simulink model "RBCM_Model"  (R2023b)
settings: Solver=FixedStepAuto  StartTime=0.0  StopTime=10.0  RelTol=1e-3
PreLoadFcn:
  | % NXP_MBDT_S32K3 callback: DO NOT REMOVE
  | mbd_s32k3.common.nxp.model_callbacks.preLoadFcn();
PostLoadFcn:
  | % NXP_MBDT_S32K3 callback: DO NOT REMOVE
  | mbd_s32k3.common.nxp.model_callbacks.postLoadFcn();
InitFcn:
  | % NXP_MBDT_S32K3 callback: DO NOT REMOVE
  | mbd_s32k3.common.nxp.model_callbacks.initFcn();
undefined symbols (not defined in the file or in its folder): AccuFanPwr_hHsd3ch2, BspdPwr_lHsd1ch2, BuzzerPwr_lHsd3ch3, DevicePwr_12v_lHsd1ch1, DevicePwr_hHsd1ch2, DrsPwr_8v_lHsd3ch1, hHsd_Diagnose_AdcBuffer, ILPwr_hHsd1ch1, lHsd_Diagnose_AdcBuffer, LoggerPwr_lHsd1ch3, PumpFan1_hHsd4ch1, PumpFan2_hHsd4ch2, PumpPwr_hHsd3ch1, RGBLED0state, TaillightPwr_lHsd3ch4, TempSensorPwr_lHsd1ch4
libraries: mbd_s32k3_io_library x127, simulink x48, canmsglib x8, mbd_s32k3_communication_library x7, mbd_s32k3_isr_library x6, mbd_s32k3_cdd_library x3, mbd_s32k3_utility_library x1
(part 1 of 9)
settings Model: DataDictionary=RBCM_Model.sldd  Creator=HUAWEI  LastModifiedBy=HUAWEI
settings SolverCC: AutoInsertRateTranBlk=on
settings DataIOCC: ExternalInput=off  InitialState=off  SaveOutput=off  SignalLogging=off  SaveTime=off
settings OptimizationCC: EnhancedBackFolding=on  PassReuseOutputArgsAs=Individual arguments  ZeroExternalMemoryAtStartup=off  ZeroInternalMemoryAtStartup=off  MaxStackSize=64  OptimizeBlockOrder=speed  DifferentSizesBufferReuse=on  OptimizationCustomize=off  EfficientTunableParamExpr=on
settings DebuggingCC: InheritedTsInSrcMsg=none  SingleTaskRateTransMsg=error  ParameterPrecisionLossMsg=none  ParameterTunabilityLossMsg=error  UnconnectedInputMsg=error  UnconnectedOutputMsg=error  UnconnectedLineMsg=error  UnknownTsInhSupMsg=error
settings HardwareCC: ProdBitPerPointer=32  ProdBitPerSizeT=32  ProdBitPerPtrDiffT=32  ProdLargestAtomicInteger=Long  ProdLargestAtomicFloat=Double  ProdWordSize=32  ProdHWDeviceType=ARM Compatible->ARM Cortex
settings SFSimCC: MATLABDynamicMemAlloc=off
settings RTWCC: Description=Embedded Coder  SystemTargetFile=ert.tlc  HardwareBoard=NXP S32K3xx  TemplateMakefile=ert_default_tmf  Toolchain=S32DS GCC  BuildConfiguration=Faster Runs  CheckMdlBeforeBuild=Warning
settings CodeAppCC: ForceParamTrailComments=on  IgnoreCustomStorageClasses=off  OperatorAnnotations=on  SimulinkDataObjDesc=on  SFDataObjDesc=on  InsertBlockDesc=on
settings ERTTargetCC: TargetLangStandard=C99 (ISO)  ExtModeTransport=1  ExtModeMexFile=ext_serial_win32_comm  ERTSrcFileBannerTemplate=mbd_s32k3_ert_code_template.cgt  ERTHdrFileBannerTemplate=mbd_s32k3_ert_code_template.cgt  ERTDataSrcFileTemplate=mbd_s32k3_ert_code_template.cgt  ERTDataHdrFileTemplate=mbd_s32k3_ert_code_template.cgt

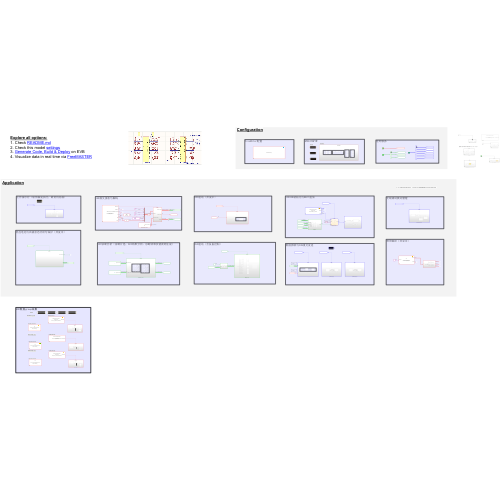
[thumbnail: Simulink's stored preview of the top-level diagram]
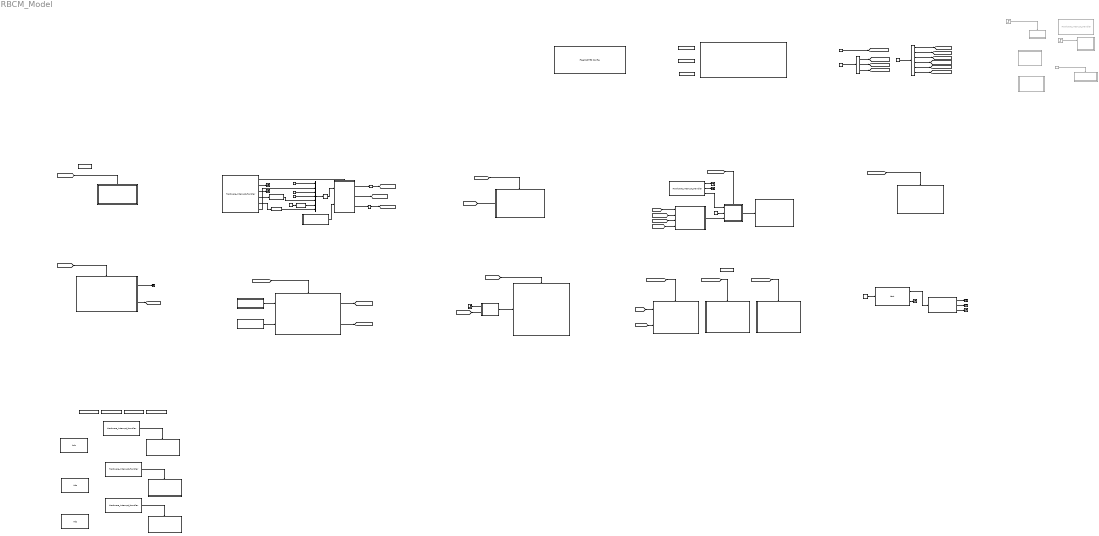
== system RBCM_Model ==
  note: Adc0Group采集
  note: ADC数据group采集
  note: 惯导解析（开发中）
  note: 初始化阶段：逐char接收，判断结束符，结束判收到字符串的ok，有则继续发
      | 通信阶段：只管发，若收转另一条任务链处理
  note: 无线调试模式管理
  note: 低压电池与自板状态分析与保护（开发中）
  note: HSD驱动（含设备控制）
  note: EC800M初始化与MQTT通信
  note: DRS驱动（开发中）
  note: Application
  note: HSD诊断分析（诊断片选、ADC结果分析、诊断结果及错误码生成）
  note: CAN报文接收与解码
  note: 工作指示灯（软件触发执行，最低优先级）
  note: 关于任务调度管理和数据传递：可以考虑采用类似DDS的数据分发服务或相关管理算法
  note: 数据抓取与CAN报文发送
  note: Explore all options:
      | 1. Check README.md
      | 2. Check this model settings
      | 3. Generate Code, Build & Deploy on EVB
      | 4. Visualize data in real time via FreeMASTER
  note: Configuration
  note: Variables
  note: Start ADC Conversions
  note: Hardware Interrupts
  note: Adc1Group采集
  note: Start ADC Conversions
  note: Hardware Interrupts
  note: Adc2Group采集
  note: Start ADC Conversions
  note: Hardware Interrupts
  note: 定时服务
  note: 初始化配置
  note: Variables
  note: Initializations
  note: FreeMster配置
  1000ms1 : simulink/Ports & Subsystems/Function-Call Generator  Priority=4  sample_time=1  numberOfIterations=1  DisallowWideOutput=off
  1000ms4 : simulink/Ports & Subsystems/Function-Call Generator  Priority=4  Commented=on  sample_time=1  numberOfIterations=1  DisallowWideOutput=off
  10ms1 : simulink/Ports & Subsystems/Function-Call Generator  Priority=4  sample_time=0.01  numberOfIterations=1  DisallowWideOutput=off
  4G通信控制状态机1 : Stateflow chart  TreatAsAtomicUnit=on
  50ms1 : simulink/Ports & Subsystems/Function-Call Generator  Priority=4  sample_time=0.05  numberOfIterations=1  DisallowWideOutput=off
  Adc1 : mbd_s32k3_io_library/Adc  api_func=Adc_StartGroupConversion  hw_unit=AdcHwUnit_0  group=Adc1Group_1  channel=hpHSD2_IS_PTD20  threshold_control=AdcThresholdControl_0  power_state=ADC_FULL_POWER  ctu_trigger=AdcHwTrigger_0  ctu_fifo_idx=0  text=<binary blob, 41534 chars, not shown>
      settings: SourceProductName=NXP Model-Based Design Toolbox for S32K3 MCUs
  Adc2 : mbd_s32k3_io_library/Adc  api_func=Adc_StartGroupConversion  hw_unit=AdcHwUnit_0  group=Adc2Group_1  channel=hpHSD2_IS_PTD20  threshold_control=AdcThresholdControl_0  power_state=ADC_FULL_POWER  ctu_trigger=AdcHwTrigger_0  ctu_fifo_idx=0  text=<binary blob, 41534 chars, not shown>
      settings: SourceProductName=NXP Model-Based Design Toolbox for S32K3 MCUs
  Adc3 : mbd_s32k3_io_library/Adc  api_func=Adc_StartGroupConversion  hw_unit=AdcHwUnit_0  group=Adc0Group_1  channel=hpHSD2_IS_PTD20  threshold_control=AdcThresholdControl_0  power_state=ADC_FULL_POWER  ctu_trigger=AdcHwTrigger_0  ctu_fifo_idx=0  text=<binary blob, 41534 chars, not shown>
      settings: SourceProductName=NXP Model-Based Design Toolbox for S32K3 MCUs
  Bitwise AND : simulink/Logic and Bit Operations/Bitwise Operator  logicop=AND  UseBitMask=on  BitMask=0x1fffffff  BitMaskRealWorld=Stored Integer
      settings: LibrarySourceBlock=|
      | simulink/Quick Insert/Logic and Bit
      | Operations/Bitwise AND
  Bus Creator1 : BusCreator  Inputs=7  OutDataTypeStr=Bus: Bus_CAN_RX_MESSAG  NonVirtualBus=on
  Constant : Constant
  Constant1 : Constant  Value=41  OutDataTypeStr=uint32
  Constant13 : Constant  Value=0  OutDataTypeStr=uint8
  Constant2 : Constant  OutDataTypeStr=uint8
  Constant4 : Constant  OutMax=[255]  OutDataTypeStr=uint8
  Constant6 : Constant  Value=0  OutDataTypeStr=uint8
  Data Store Memory1 : DataStoreMemory  DataStoreName=Adc0Group1_ResultBuffer  ReadBeforeWriteMsg=warning  WriteAfterWriteMsg=warning  WriteAfterReadMsg=warning  InitialValue=[0, 0, 0, 0, 0, 0]  ShowAdditionalParam=off  OutDataTypeStr=uint16
  Data Store Memory2 : DataStoreMemory  DataStoreName=Temp_AdcBuffer  WriteAfterWriteMsg=warning  ShowAdditionalParam=off  OutDataTypeStr=uint16
  Data Store Memory3 : DataStoreMemory  DataStoreName=can_id  ReadBeforeWriteMsg=warning  WriteAfterWriteMsg=warning  WriteAfterReadMsg=warning  ShowAdditionalParam=off  OutDataTypeStr=uint32
  Data Store Memory4 : DataStoreMemory  DataStoreName=Bats_Monitor_AdcBuffer  WriteAfterWriteMsg=warning  InitialValue=[0 0]  ShowAdditionalParam=off  OutDataTypeStr=uint16
  Data Store Memory5 : DataStoreMemory  DataStoreName=hHsd_Diagnose_AdcBuffer  WriteAfterWriteMsg=warning  InitialValue=[0 0 0 0 0 0]  ShowAdditionalParam=off  OutDataTypeStr=uint16
  Data Store Memory6 : DataStoreMemory  DataStoreName=lHsd_Diagnose_AdcBuffer  WriteAfterWriteMsg=warning  InitialValue=[0 0 0 0 0]  ShowAdditionalParam=off  OutDataTypeStr=uint16
  Data Store Memory7 : DataStoreMemory  DataStoreName=Adc1Group1_ResultBuffer  ReadBeforeWriteMsg=warning  WriteAfterWriteMsg=warning  WriteAfterReadMsg=warning  InitialValue=[0, 0, 0]  ShowAdditionalParam=off  OutDataTypeStr=uint16
  Data Store Memory8 : DataStoreMemory  DataStoreName=Adc2Group1_ResultBuffer  ReadBeforeWriteMsg=warning  WriteAfterWriteMsg=warning  WriteAfterReadMsg=warning  InitialValue=[0, 0, 0, 0, 0]  ShowAdditionalParam=off  OutDataTypeStr=uint16
  Data Type Conversion2 : DataTypeConversion  OutDataTypeStr=double  SaturateOnIntegerOverflow=off  RndMeth=Floor
  Delay : Delay  DelayLength=1
  FreeMASTER Config : mbd_s32k3_utility_library/FreeMASTER blocks/FreeMASTER Config  connection_type=Serial  instance=LPUART_6  baudrate=115200  isr_prio=5  cantxid=0x7aa  cantxidext=on  cantxobj=5  canrxid=0x7aa  canrxidext=on  canrxobj=5  mode=Short Interrupt  scope_use=1  scope_max_vars=8  automatic_buff_size=on  buff_size=255  default_rfifo_size=on  rfifo_size=32  text=This peripheral is not configured in the project associated to the model.
      settings: SourceProductName=NXP Model-Based Design Toolbox for S32K3 MCUs
  Function-Call Split : FunctionCallSplit  IconShape=distinctive  NumOutputPorts=6  OutputPortLayout=default
  Function-Call Split1 : FunctionCallSplit  IconShape=distinctive  NumOutputPorts=3  OutputPortLayout=default
  HSD诊断分析子系统 : Subsystem
  HSD诊断数据抓取与发送(不启用) : Subsystem  Commented=on
  HSD驱动子系统 : Subsystem
  Hardware_Interrupt_Handler : mbd_s32k3_isr_library/Hardware_Interrupt_Handler  blockCbk=0  irqGroup=Uart  irqHandlers=MBDT_Uart_Callback  irqSim=off  text=<binary blob, 5810 chars, not shown>
      settings: SourceProductName=NXP Model-Based Design Toolbox for S32K3 MCUs
  Hardware_Interrupt_Handler1 : mbd_s32k3_isr_library/Hardware_Interrupt_Handler  blockCbk=0  irqGroup=Adc  irqHandlers=Adc_Adc0Group1Notification  irqSim=off  text=<binary blob, 41534 chars, not shown>
      settings: SourceProductName=NXP Model-Based Design Toolbox for S32K3 MCUs
  Hardware_Interrupt_Handler2 : mbd_s32k3_isr_library/Hardware_Interrupt_Handler  blockCbk=0  irqGroup=Adc  irqHandlers=Adc_Adc1Group1Notification  irqSim=off  text=<binary blob, 41534 chars, not shown>
      settings: SourceProductName=NXP Model-Based Design Toolbox for S32K3 MCUs
  Hardware_Interrupt_Handler4 : mbd_s32k3_isr_library/Hardware_Interrupt_Handler  blockCbk=0  irqGroup=Can  irqHandlers=CanIf_RxIndication  irqSim=off  text=|
      | CanConfigSet - CanConfigSet 
      | CanConfigSet/CanController - CanController_0 
      | CanConfigSet/CanController_0/CanAutoBusOffRecovery - false 
      | CanConfigSet/CanController_0/CanBusoffProcessing - POLLING 
      | CanConfigSet/CanController_0/CanControllerActivation - true 
      | CanConfigSet/CanController_0/CanControllerBaseAddress - 0 
      | CanConfigSet/CanController_0/CanControllerBaudrateConfig - CanControllerBaudrateConfig_0 
      | CanConfigSet/CanController_0/CanControllerBaudrateConfig_0/CanAdvancedSetting - false 
      | CanConfigSet/CanController_0/CanControllerBaudrateConfig_0/CanBaudrateTypeSuport - NORMAL_CBT 
      | CanConfigSet/CanController_0/CanControllerBaudrateConfig_0/CanBusLength - 40 
      | CanConfigSet/CanController_0/CanControllerBaudrateConfig_0/CanControllerBaudRate - 500.0 
      | CanConfigSet/CanController_0/CanControllerBaudrateConfig_0/CanControllerBaudRateConfigID - 0 
      | CanConfigSet/CanController_0/CanControllerBaudrateConfig_0/CanControllerFdBaudrateConfig - CanControllerFdBaudrateConfig 
      | CanConfigSet/CanController_0/CanControllerBaudrateConfig_0/CanControllerFdBaudrateConfig/CanControllerFdBaudRate - 2000 
      | CanConfigSet/CanController_0/CanControllerBaudrateConfig_0/CanControllerFdBaudrateConfig/CanControllerFdPrescaller - 2 
      | CanConfigSet/CanController_0/CanControllerBaudrateConfig_0/CanControllerFdBaudrateConfig/CanControllerFdSyncSeg - 1 
      | CanConfigSet/CanController_0/CanControllerBaudrateConfig_0/CanControllerFdBaudrateConfig/CanControllerPrescallerAlternateFd - 1 
      | CanConfigSet/CanController_0/CanControllerBaudrateConfig_0/CanControllerFdBaudrateConfig/CanControllerPropSeg - 5 
      | CanConfigSet/CanController_0/CanControllerBaudrateConfig_0/CanControllerFdBaudrateConfig/CanControllerSeg1 - 2 
      | CanConfigSet/CanController_0/CanControllerBaudrateConfig_0/CanControllerFdBaudrateConfig/CanControllerSeg2 - 2 
      | CanConfigSet/CanController_0/CanControllerBaudrateConfig_0/CanControllerFdBaudrateConfig/CanControllerSyncJumpWidth - 2 
      | CanConfigSet/CanController_0/CanControllerBaudrateConfig_0/CanControllerFdBaudrateConfig/CanControllerTxBitRateSwitch - true 
      | CanConfigSet/CanController_0/CanControllerBaudrateConfig_0/CanControllerFdBaudrateConfig/Index - 0 
      | CanConfigSet/CanController_0/CanControllerBaudrateConfig_0/CanControllerPrescaller - 2 
      | CanConfigSet/CanController_0/CanControllerBaudrateConfig_0/CanControllerPrescallerAlternate - 10 
      | CanConfigSet/CanController_0/CanControllerBaudrateConfig_0/CanControllerPropSeg - 11 
      | CanConfigSet/CanController_0/CanControllerBaudrateConfig_0/CanControllerSeg1 - 18 
      | CanConfigSet/CanController_0/CanControllerBaudrateConfig_0/CanControllerSeg2 - 10 
      | CanConfigSet/CanController_0/CanControllerBaudrateConfig_0/CanControllerSyncJumpWidth - 10 
      | CanConfigSet/CanController_0/CanControllerBaudrateConfig_0/CanControllerSyncSeg - 1 
      | CanConfigSet/CanController_0/CanControllerBaudrateConfig_0/CanPropDelayTranceiver - 150.0 
      | CanConfigSet/CanController_0/CanControllerBaudrateConfig_0/CanTxArbitrationStartDelay - 12 
      | CanConfigSet/CanController_0/CanControllerBaudrateConfig_0/Index - 0 
      | CanConfigSet/CanController_0/CanControllerDefaultBaudrate - /Can_43_FLEXCAN/Can/CanConfigSet/CanController_0/CanControllerBaudrateConfig_0 
      | CanConfigSet/CanController_0/CanControllerEdgeFilter - false 
      | CanConfigSet/CanController_0/CanControllerFdISO - true 
      | CanConfigSet/CanController_0/CanControllerId - 0 
      | CanConfigSet/CanController_0/CanControllerPrExcEn - false 
      | CanConfigSet/CanController_0/CanCpuClockRef - /Mcu/Mcu/McuModuleConfiguration/McuClockSettingConfig_0/FLEXCAN_PE_CLK0_2 
      | CanConfigSet/CanController_0/CanCpuClockRefAlternate - /Mcu/Mcu/McuModuleConfiguration/McuClockSettingConfig_0/FLEXCAN_PE_CLK0_2 
      | CanConfigSet/CanController_0/CanHwChannel - FLEXCAN_0 
      | CanConfigSet/CanController_0/CanLoopBackMode - false 
      | CanConfigSet/CanController_0/CanRamBlock - CanRamBlock 
      | CanConfigSet/CanController_0/CanRamBlock/CanRamBlockUnified - CanRamBlockUnified 
      | CanConfigSet/CanController_0/CanRamBlock/CanRamBlockUnified/CanBlockUnifiedPayloadLength - CAN_16_BYTES_PAYLOAD 
      | CanConfigSet/CanController_0/CanRamBlock/Choice - CanRamBlockUnified 
      | CanConfigSet/CanController_0/CanRamBlock/Index - 0 
      | CanConfigSet/CanController_0/CanRxFiFo - CanRxFiFo 
      | CanConfigSet/CanController_0/CanRxFiFo/CanEnhanceFiFo - CanRxFiFo 
      | CanConfigSet/CanController_0/CanRxFiFo/CanRxFiFo/CanEnhanceFiFoDmaEnable - false 
      | CanConfigSet/CanController_0/CanRxFiFo/CanRxFiFo/CanEnhancedSchemeType - MASK_FILTER_SCHEME 
      | CanConfigSet/CanController_0/CanRxFiFo/CanRxFiFo/CanFiFoDmaErrorNotif - NULL_PTR 
      | CanConfigSet/CanController_0/CanRxFiFo/CanRxFiFo/CanFiFoOverflowNotif - MBDT_FlexCAN0_FifoOverflowNotif 
      | CanConfigSet/CanController_0/CanRxFiFo/CanRxFiFo/NumberMBTransferDMA - 1 
      | CanConfigSet/CanController_0/CanRxFiFo/Choice - CanEnhanceFiFo 
      | CanConfigSet/CanController_0/CanRxFiFo/Index - 0 
      | CanConfigSet/CanController_0/CanRxProcessing - MIXED 
      | CanConfigSet/CanController_0/CanTrippleSamplingEnable - false 
      | CanConfigSet/CanController_0/CanTxProcessing - MIXED 
      | CanConfigSet/CanController_0/CanWakeupFunctionalityAPI - false 
      | CanConfigSet/CanController_0/CanWakeupProcessing - POLLING 
      | CanConfigSet/CanController_0/CanWakeupSupport - false 
      | CanConfigSet/CanController_0/Index - 0 
      | CanConfigSet/CanHardwareObject - CanHardwareObject_Can0_Rx_Ext_Interrupt CanHardwareObject_Can0_Rx_FIFO CanHardwareObject_Can0_Rx_Std_Polling CanHardwareObject_Can0_Tx_Interrupt CanHardwareObject_Can0_Tx_Polling 
      | CanConfigSet/CanHardwareObject_Can0_Rx_Ext_Interrupt/CanControllerRef - /Can_43_FLEXCAN/Can/CanConfigSet/CanController_0 
      | CanConfigSet/CanHardwareObject_Can0_Rx_Ext_Interrupt/CanHandleType - BASIC 
      | CanConfigSet/CanHardwareObject_Can0_Rx_Ext_Interrupt/CanHardwareObjectUsesPolling - false 
      | CanConfigSet/CanHardwareObject_Can0_Rx_Ext_Interrupt/CanHwFilter - CanHwFilter_0 
      | CanConfigSet/CanHardwareObject_Can0_Rx_Ext_Interrupt/CanHwFilter_0/CanHwFilterCode - 0 
      | CanConfigSet/CanHardwareObject_Can0_Rx_Ext_Interrupt/CanHwFilter_0/CanHwFilterMask - 0 
      | CanConfigSet/CanHardwareObject_Can0_Rx_Ext_Interrupt/CanHwFilter_0/Index - 0 
      | CanConfigSet/CanHardwareObject_Can0_Rx_Ext_Interrupt/CanHwObjectCount - 1 
      | CanConfigSet/CanHardwareObject_Can0_Rx_Ext_Interrupt/CanIdType - EXTENDED 
      | CanConfigSet/CanHardwareObject_Can0_Rx_Ext_Interrupt/CanObjectId - 2 
      | CanConfigSet/CanHardwareObject_Can0_Rx_Ext_Interrupt/CanObjectType - RECEIVE 
      | CanConfigSet/CanHardwareObject_Can0_Rx_Ext_Interrupt/Index - 2 
      | CanConfigSet/CanHardwareObject_Can0_Rx_FIFO/CanControllerRef - /Can_43_FLEXCAN/Can/CanConfigSet/CanController_0 
      | CanConfigSet/CanHardwareObject_Can0_Rx_FIFO/CanHandleType - BASIC 
      | CanConfigSet/CanHardwareObject_Can0_Rx_FIFO/CanHardwareObjectUsesPolling - false 
      | CanConfigSet/CanHardwareObject_Can0_Rx_FIFO/CanHwFilter - CanHwFilter_0 CanHwFilter_1 CanHwFilter_2 CanHwFilter_3 CanHwFilter_4 CanHwFilter_5 CanHwFilter_6 CanHwFilter_7 
      | CanConfigSet/CanHardwareObject_Can0_Rx_FIFO/CanHwFilter_0/CanHwFilterCode - 1008 
      | CanConfigSet/CanHardwareObject_Can0_Rx_FIFO/CanHwFilter_0/CanHwFilterMask - 536870911 
      | CanConfigSet/CanHardwareObject_Can0_Rx_FIFO/CanHwFilter_0/Index - 0 
      | CanConfigSet/CanHardwareObject_Can0_Rx_FIFO/CanHwFilter_1/CanHwFilterCode - 1009 
      | CanConfigSet/CanHardwareObject_Can0_Rx_FIFO/CanHwFilter_1/CanHwFilterMask - 536870911 
      | CanConfigSet/CanHardwareObject_Can0_Rx_FIFO/CanHwFilter_1/Index - 1 
      | CanConfigSet/CanHardwareObject_Can0_Rx_FIFO/CanHwFilter_2/CanHwFilterCode - 1010 
      | CanConfigSet/CanHardwareObject_Can0_Rx_FIFO/CanHwFilter_2/CanHwFilterMask - 536870911 
      | CanConfigSet/CanHardwareObject_Can0_Rx_FIFO/CanHwFilter_2/Index - 2 
      | CanConfigSet/CanHardwareObject_Can0_Rx_FIFO/CanHwFilter_3/CanHwFilterCode - 1011 
      | CanConfigSet/CanHardwareObject_Can0_Rx_FIFO/CanHwFilter_3/CanHwFilterMask - 536870911 
      | CanConfigSet/CanHardwareObject_Can0_Rx_FIFO/CanHwFilter_3/Index - 3 
      | CanConfigSet/CanHardwareObject_Can0_Rx_FIFO/CanHwFilter_4/CanHwFilterCode - 1012 
      | CanConfigSet/CanHardwareObject_Can0_Rx_FIFO/CanHwFilter_4/CanHwFilterMask - 536870911 
      | CanConfigSet/CanHardwareObject_Can0_Rx_FIFO/CanHwFilter_4/Index - 4 
      | CanConfigSet/CanHardwareObject_Can0_Rx_FIFO/CanHwFilter_5/CanHwFilterCode - 1013 
      | CanConfigSet/CanHardwareObject_Can0_Rx_FIFO/CanHwFilter_5/CanHwFilterMask - 536870911 
      | CanConfigSet/CanHardwareObject_Can0_Rx_FIFO/CanHwFilter_5/Index - 5 
      | CanConfigSet/CanHardwareObject_Can0_Rx_FIFO/CanHwFilter_6/CanHwFilterCode - 1014 
      | CanConfigSet/CanHardwareObject_Can0_Rx_FIFO/CanHwFilter_6/CanHwFilterMask - 536870911 
      | CanConfigSet/CanHardwareObject_Can0_Rx_FIFO/CanHwFilter_6/Index - 6 
      | CanConfigSet/CanHardwareObject_Can0_Rx_FIFO/CanHwFilter_7/CanHwFilterCode - 1015 
      | CanConfigSet/CanHardwareObject_Can0_Rx_FIFO/CanHwFilter_7/CanHwFilterMask - 536870911 
      | CanConfigSet/CanHardwareObject_Can0_Rx_FIFO/CanHwFilter_7/Index - 7 
      | CanConfigSet/CanHardwareObject_Can0_Rx_FIFO/CanHwObjectCount - 6 
      | CanConfigSet/CanHardwareObject_Can0_Rx_FIFO/CanIdType - EXTENDED 
      | CanConfigSet/CanHardwareObject_Can0_Rx_FIFO/CanObjectId - 0 
      | CanConfigSet/CanHardwareObject_Can0_Rx_FIFO/CanObjectType - RECEIVE 
      | CanConfigSet/CanHardwareObject_Can0_Rx_FIFO/Index - 0 
      | CanConfigSet/CanHardwareObject_Can0_Rx_Std_Polling/CanControllerRef - /Can_43_FLEXCAN/Can/CanConfigSet/CanController_0 
      | CanConfigSet/CanHardwareObject_Can0_Rx_Std_Polling/CanHandleType - BASIC 
      | CanConfigSet/CanHardwareObject_Can0_Rx_Std_Polling/CanHardwareObjectUsesPolling - true 
      | CanConfigSet/CanHardwareObject_Can0_Rx_Std_Polling/CanHwFilter - CanHwFilter_0 
      | CanConfigSet/CanHardwareObject_Can0_Rx_Std_Polling/CanHwFilter_0/CanHwFilterCode - 0 
      | CanConfigSet/CanHardwareObject_Can0_Rx_Std_Polling/CanHwFilter_0/CanHwFilterMask - 0 
      | CanConfigSet/CanHardwareObject_Can0_Rx_Std_Polling/CanHwFilter_0/Index - 0 
      | CanConfigSet/CanHardwareObject_Can0_Rx_Std_Polling/CanHwObjectCount - 1 
      | CanConfigSet/CanHardwareObject_Can0_Rx_Std_Polling/CanIdType - STANDARD 
      | CanConfigSet/CanHardwareObject_Can0_Rx_Std_Polling/CanMainFunctionRWPeriodRef - /Can_43_FLEXCAN/Can/CanGeneral/CanMainFunctionRWPeriods_0 
      | CanConfigSet/CanHardwareObject_Can0_Rx_Std_Polling/CanObjectId - 1 
      | CanConfigSet/CanHardwareObject_Can0_Rx_Std_Polling/CanObjectType - RECEIVE 
      | CanConfigSet/CanHardwareObject_Can0_Rx_Std_Polling/Index - 1 
      | CanConfigSet/CanHardwareObject_Can0_Tx_Interrupt/CanControllerRef - /Can_43_FLEXCAN/Can/CanConfigSet/CanController_0 
      | CanConfigSet/CanHardwareObject_Can0_Tx_Interrupt/CanHandleType - BASIC 
      | CanConfigSet/CanHardwareObject_Can0_Tx_Interrupt/CanHardwareObjectUsesPolling - false 
      | CanConfigSet/CanHardwareObject_Can0_Tx_Interrupt/CanHwObjectCount - 1 
      | CanConfigSet/CanHardwareObject_Can0_Tx_Interrupt/CanIdType - MIXED 
      | CanConfigSet/CanHardwareObject_Can0_Tx_Interrupt/CanObjectId - 4 
      | CanConfigSet/CanHardwareObject_Can0_Tx_Interrupt/CanObjectType - TRANSMIT 
      | CanConfigSet/CanHardwareObject_Can0_Tx_Interrupt/Index - 4 
      | CanConfigSet/CanHardwareObject_Can0_Tx_Polling/CanControllerRef - /Can_43_FLEXCAN/Can/CanConfigSet/CanController_0 
      | CanConfigSet/CanHardwareObject_Can0_Tx_Polling/CanHandleType - BASIC 
      | CanConfigSet/CanHardwareObject_Can0_Tx_Polling/CanHardwareObjectUsesPolling - true 
      | CanConfigSet/CanHardwareObject_Can0_Tx_Polling/CanHwObjectCount - 1 
      | CanConfigSet/CanHardwareObject_Can0_Tx_Polling/CanIdType - MIXED 
      | CanConfigSet/CanHardwareObject_Can0_Tx_Polling/CanMainFunctionRWPeriodRef - /Can_43_FLEXCAN/Can/CanGeneral/CanMainFunctionRWPeriods_0 
      | CanConfigSet/CanHardwareObject_Can0_Tx_Polling/CanObjectId - 3 
      | CanConfigSet/CanHardwareObject_Can0_Tx_Polling/CanObjectType - TRANSMIT 
      | CanConfigSet/CanHardwareObject_Can0_Tx_Polling/Index - 3 
      | CanGeneral - CanGeneral 
      | CanGeneral/CanApiEnableMbAbort - true 
      | CanGeneral/CanDevErrorDetect - true 
      | CanGeneral/CanEnableDualClockMode - false 
      | CanGeneral/CanEnableSecurityEventReporting - false 
      | CanGeneral/CanEnableUserModeSupport - false 
      | CanGeneral/CanGlobalTimeSupport - false 
      | CanGeneral/CanIndex - 0 
      | CanGeneral/CanMBCountExtensionSupport - false 
      | CanGeneral/CanMainFunctionModePeriod - 0.001 
      | CanGeneral/CanMainFunctionRWPeriods - CanMainFunctionRWPeriods_0 
      | CanGeneral/CanMainFunctionRWPeriods_0/CanMainFunctionPeriod - 0.001 
      | CanGeneral/CanMainFunctionRWPeriods_0/Index - 0 
      | CanGeneral/CanMultiPartitionSupport - false 
      | CanGeneral/CanMultiplexedTransmission - true 
      | CanGeneral/CanSetBaudrateApi - true 
      | CanGeneral/CanTimeoutDuration - 1.0 
      | CanGeneral/CanTimeoutMethod - OSIF_COUNTER_DUMMY 
      | CanGeneral/CanVersionInfoApi - true 
      | CommonPublishedInformation - CommonPublishedInformation 
      | CommonPublishedInformation/ArReleaseMajorVersion - 4 
      | CommonPublishedInformation/ArReleaseMinorVersion - 7 
      | CommonPublishedInformation/ArReleaseRevisionVersion - 0 
      | CommonPublishedInformation/ModuleId - 80 
      | CommonPublishedInformation/SwMajorVersion - 3 
      | CommonPublishedInformation/SwMinorVersion - 0 
      | CommonPublishedInformation/SwPatchVersion - 0 
      | CommonPublishedInformation/VendorApiInfix - FLEXCAN 
      | CommonPublishedInformation/VendorId - 43 
      | IMPLEMENTATION-CONFIG-VARIANT - VARIANT-POST-BUILD 
      | POST_BUILD_VARIANT_USED - true
      settings: SourceProductName=NXP Model-Based Design Toolbox for S32K3 MCUs
  Hardware_Interrupt_Handler5 : mbd_s32k3_isr_library/Hardware_Interrupt_Handler  blockCbk=0  irqGroup=Adc  irqHandlers=Adc_Adc2Group1Notification  irqSim=off  text=<binary blob, 41534 chars, not shown>
      settings: SourceProductName=NXP Model-Based Design Toolbox for S32K3 MCUs
  Hardware_Interrupt_Handler6 : mbd_s32k3_isr_library/Hardware_Interrupt_Handler  Commented=on  blockCbk=0  irqGroup=Pwm  irqHandlers=PwmChannel_0_Callback  irqSim=off  text=|
      | CommonPublishedInformation - CommonPublishedInformation Pwm 
      | CommonPublishedInformation/ArReleaseMajorVersion - 4 
      | CommonPublishedInformation/ArReleaseMinorVersion - 4 
      | CommonPublishedInformation/ArReleaseRevisionVersion - 0 
      | CommonPublishedInformation/ModuleId - 121 
      | CommonPublishedInformation/SwMajorVersion - 2 
      | CommonPublishedInformation/SwMinorVersion - 0 
      | CommonPublishedInformation/SwPatchVersion - 0 
      | CommonPublishedInformation/VendorId - 43 
      | IMPLEMENTATION-CONFIG-VARIANT - VARIANT-POST-BUILD 
      | POST_BUILD_VARIANT_USED - true 
      | PwmChannel - PwmChannel_0 PwmChannel_1 PwmChannel_2 PwmChannel_3 PwmChannel_4 PwmChannel_5 PwmChannel_6 PwmChannel_7 PwmChannel_8 
      | PwmChannel_0/Index - 0 
      | PwmChannel_0/PwmChannelId - 0 
      | PwmChannel_0/PwmDutycycleDefault - 2048 
      | PwmChannel_0/PwmHwChannel - /Pwm/Pwm/PwmChannelConfigSet/PwmEmios_0/PwmEmiosChannels_9 
      | PwmChannel_0/PwmIdleState - PWM_LOW 
      | PwmChannel_0/PwmMcuClockReferencePoint - /Mcu/Mcu/McuModuleConfiguration/McuClockSettingConfig_0/CORE_CLK 
      | PwmChannel_0/PwmNotification - PwmChannel_0_Callback 
      | PwmChannel_0/PwmPeriodDefault - 16000.0 
      | PwmChannel_0/PwmPeriodInTicks - true 
      | PwmChannel_0/PwmPolarity - PWM_HIGH 
      | PwmChannel_1/Index - 1 
      | PwmChannel_1/PwmChannelId - 1 
      | PwmChannel_1/PwmDutycycleDefault - 2048 
      | PwmChannel_1/PwmHwChannel - /Pwm/Pwm/PwmChannelConfigSet/PwmEmios_0/PwmEmiosChannels_17 
      | PwmChannel_1/PwmIdleState - PWM_LOW 
      | PwmChannel_1/PwmMcuClockReferencePoint - /Mcu/Mcu/McuModuleConfiguration/McuClockSettingConfig_0/CORE_CLK 
      | PwmChannel_1/PwmNotification - PwmChannel_1_Callback 
      | PwmChannel_1/PwmPeriodDefault - 16000.0 
      | PwmChannel_1/PwmPeriodInTicks - true 
      | PwmChannel_1/PwmPolarity - PWM_HIGH 
      | PwmChannel_2/Index - 2 
      | PwmChannel_2/PwmChannelId - 2 
      | PwmChannel_2/PwmDutycycleDefault - 0 
      | PwmChannel_2/PwmHwChannel - /Pwm/Pwm/PwmChannelConfigSet/PwmEmios_1/PwmEmiosChannels_19 
      | PwmChannel_2/PwmIdleState - PWM_LOW 
      | PwmChannel_2/PwmMcuClockReferencePoint - /Mcu/Mcu/McuModuleConfiguration/McuClockSettingConfig_0/CORE_CLK 
      | PwmChannel_2/PwmNotification - PwmChannel_2_Callback 
      | PwmChannel_2/PwmPeriodDefault - 16000.0 
      | PwmChannel_2/PwmPeriodInTicks - true 
      | PwmChannel_2/PwmPolarity - PWM_HIGH 
      | PwmChannel_3/Index - 3 
      | PwmChannel_3/PwmChannelId - 3 
      | PwmChannel_3/PwmDutycycleDefault - 0 
      | PwmChannel_3/PwmHwChannel - /Pwm/Pwm/PwmChannelConfigSet/PwmEmios_1/PwmEmiosChannels_20 
      | PwmChannel_3/PwmIdleState - PWM_LOW 
      | PwmChannel_3/PwmMcuClockReferencePoint - /Mcu/Mcu/McuModuleConfiguration/McuClockSettingConfig_0/CORE_CLK 
      | PwmChannel_3/PwmNotification - PwmChannel_3_Callback 
      | PwmChannel_3/PwmPeriodDefault - 16000.0 
      | PwmChannel_3/PwmPeriodInTicks - true 
      | PwmChannel_3/PwmPolarity - PWM_HIGH 
      | PwmChannel_4/Index - 4 
      | PwmChannel_4/PwmChannelId - 4 
      | PwmChannel_4/PwmDutycycleDefault - 0 
      | PwmChannel_4/PwmHwChannel - /Pwm/Pwm/PwmChannelConfigSet/PwmEmios_1/PwmEmiosChannels_0 
      | PwmChannel_4/PwmIdleState - PWM_LOW 
      | PwmChannel_4/PwmMcuClockReferencePoint - /Mcu/Mcu/McuModuleConfiguration/McuClockSettingConfig_0/CORE_CLK 
      | PwmChannel_4/PwmNotification - PwmChannel_4_Callback 
      | PwmChannel_4/PwmPeriodDefault - 16000.0 
      | PwmChannel_4/PwmPeriodInTicks - true 
      | PwmChannel_4/PwmPolarity - PWM_HIGH 
      | PwmChannel_5/Index - 5 
      | PwmChannel_5/PwmChannelId - 5 
      | PwmChannel_5/PwmDutycycleDefault - 0 
      | PwmChannel_5/PwmHwChannel - /Pwm/Pwm/PwmChannelConfigSet/PwmEmios_1/PwmEmiosChannels_1 
      | PwmChannel_5/PwmIdleState - PWM_LOW 
      | PwmChannel_5/PwmMcuClockReferencePoint - /Mcu/Mcu/McuModuleConfiguration/McuClockSettingConfig_0/CORE_CLK 
      | PwmChannel_5/PwmNotification - PwmChannel_5_Callback 
      | PwmChannel_5/PwmPeriodDefault - 16000.0 
      | PwmChannel_5/PwmPeriodInTicks - true 
      | PwmChannel_5/PwmPolarity - PWM_HIGH 
      | PwmChannel_6/Index - 6 
      | PwmChannel_6/PwmChannelId - 6 
      | PwmChannel_6/PwmDutycycleDefault - 0 
      | PwmChannel_6/PwmHwChannel - /Pwm/Pwm/PwmChannelConfigSet/PwmEmios_1/PwmEmiosChannels_21 
      | PwmChannel_6/PwmIdleState - PWM_LOW 
      | PwmChannel_6/PwmMcuClockReferencePoint - /Mcu/Mcu/McuModuleConfiguration/McuClockSettingConfig_0/CORE_CLK 
      | PwmChannel_6/PwmNotification - PwmChannel_6_Callback 
      | PwmChannel_6/PwmPeriodDefault - 16000.0 
      | PwmChannel_6/PwmPeriodInTicks - true 
      | PwmChannel_6/PwmPolarity - PWM_HIGH 
      | PwmChannel_7/Index - 7 
      | PwmChannel_7/PwmChannelId - 7 
      | PwmChannel_7/PwmDutycycleDefault - 0 
      | PwmChannel_7/PwmHwChannel - /Pwm/Pwm/PwmChannelConfigSet/PwmEmios_1/PwmEmiosChannels_22 
      | PwmChannel_7/PwmIdleState - PWM_LOW 
      | PwmChannel_7/PwmMcuClockReferencePoint - /Mcu/Mcu/McuModuleConfiguration/McuClockSettingConfig_0/CORE_CLK 
      | PwmChannel_7/PwmNotification - PwmChannel_7_Callback 
      | PwmChannel_7/PwmPeriodDefault - 16000.0 
      | PwmChannel_7/PwmPeriodInTicks - true 
      | PwmChannel_7/PwmPolarity - PWM_HIGH 
      | PwmChannel_8/Index - 8 
      | PwmChannel_8/PwmChannelId - 8 
      | PwmChannel_8/PwmDutycycleDefault - 0 
      | PwmChannel_8/PwmHwChannel - /Pwm/Pwm/PwmChannelConfigSet/PwmEmios_2/PwmEmiosChannels_7 
      | PwmChannel_8/PwmIdleState - PWM_LOW 
      | PwmChannel_8/PwmMcuClockReferencePoint - /Mcu/Mcu/McuModuleConfiguration/McuClockSettingConfig_0/CORE_CLK 
      | PwmChannel_8/PwmNotification - PwmChannel_8_Callback 
      | PwmChannel_8/PwmPeriodDefault - 40000 
      | PwmChannel_8/PwmPeriodInTicks - true 
      | PwmChannel_8/PwmPolarity - PWM_HIGH 
      | PwmConfigurationOfOptApiServices - PwmConfigurationOfOptApiServices 
      | PwmConfigurationOfOptApiServices/PwmDeInitApi - true 
      | PwmConfigurationOfOptApiServices/PwmEmiosFastUpdateApi - true 
      | PwmConfigurationOfOptApiServices/PwmEnableMaskOutputs - false 
      | PwmConfigurationOfOptApiServices/PwmGetChannelStateApi - true 
      | PwmConfigurationOfOptApiServices/PwmGetOutputState - true 
      | PwmConfigurationOfOptApiServices/PwmSetChannelDeadTime - true 
      | PwmConfigurationOfOptApiServices/PwmSetChannelOutputApi - true 
      | PwmConfigurationOfOptApiServices/PwmSetCounterBusApi - true 
      | PwmConfigurationOfOptApiServices/PwmSetDutyCycle - true 
      | PwmConfigurationOfOptApiServices/PwmSetDutyCycle_NoUpdate - false 
      | PwmConfigurationOfOptApiServices/PwmSetDutyPhaseShift - false 
      | PwmConfigurationOfOptApiServices/PwmSetOutputToIdle - true 
      | PwmConfigurationOfOptApiServices/PwmSetPeriodAndDuty - true 
      | PwmConfigurationOfOptApiServices/PwmSetPeriodAndDuty_NoUpdate - false 
      | PwmConfigurationOfOptApiServices/PwmSetTriggerDelayApi - true 
      | PwmConfigurationOfOptApiServices/PwmVersionInfoApi - true 
      | PwmEmios - PwmEmios_0 PwmEmios_1 PwmEmios_2 
      | PwmEmios_0/Index - 0 
      | PwmEmios_0/PwmEmiosChannels - PwmEmiosChannels_17 PwmEmiosChannels_9 
      | PwmEmios_0/PwmEmiosChannels_17/EmiosChCounterBus - EMIOS_PWM_IP_BUS_A 
      | PwmEmios_0/PwmEmiosChannels_17/EmiosChDeadtime - 0 
      | PwmEmios_0/PwmEmiosChannels_17/EmiosChFlagGeneration - Trailing_Edge 
      | PwmEmios_0/PwmEmiosChannels_17/EmiosChFreeze - false 
      | PwmEmios_0/PwmEmiosChannels_17/EmiosChId - CH_17 
      | PwmEmios_0/PwmEmiosChannels_17/EmiosChInterrupt - EMIOS_PWM_IP_INTERRUPT_REQUEST 
      | PwmEmios_0/PwmEmiosChannels_17/EmiosChMode - EMIOS_PWM_IP_MODE_OPWMB 
      | PwmEmios_0/PwmEmiosChannels_17/EmiosChOutputDisable - EMIOS_PWM_IP_OUTPUT_DISABLE_NONE 
      | PwmEmios_0/PwmEmiosChannels_17/EmiosChPhaseShift - 0 
      | PwmEmios_0/PwmEmiosChannels_17/EmiosChPrescaler - EMIOS_PWM_IP_CLOCK_DIV_2 
      | PwmEmios_0/PwmEmiosChannels_17/EmiosChPrescalerAlternate - EMIOS_PWM_IP_CLOCK_DIV_1 
      | PwmEmios_0/PwmEmiosChannels_17/EmiosChPrescalerSource - EMIOS_PWM_IP_PS_SRC_MODULE_CLOCK 
      | PwmEmios_0/PwmEmiosChannels_17/EmiosChTrigger - 0 
      | PwmEmios_0/PwmEmiosChannels_17/Index - 1 
      | PwmEmios_0/PwmEmiosChannels_17/PwmEmiosBusRef - /Mcl/Mcl/MclConfig/EmiosCommon_0/EmiosMclMasterBus_0 
      | PwmEmios_0/PwmEmiosChannels_9/EmiosChCounterBus - EMIOS_PWM_IP_BUS_A 
      | PwmEmios_0/PwmEmiosChannels_9/EmiosChDeadtime - 0 
      | PwmEmios_0/PwmEmiosChannels_9/EmiosChFlagGeneration - Trailing_Edge 
      | PwmEmios_0/PwmEmiosChannels_9/EmiosChFreeze - false 
      | PwmEmios_0/PwmEmiosChannels_9/EmiosChId - CH_9 
      | PwmEmios_0/PwmEmiosChannels_9/EmiosChInterrupt - EMIOS_PWM_IP_INTERRUPT_REQUEST 
      | PwmEmios_0/PwmEmiosChannels_9/EmiosChMode - EMIOS_PWM_IP_MODE_OPWMB 
      | PwmEmios_0/PwmEmiosChannels_9/EmiosChOutputDisable - EMIOS_PWM_IP_OUTPUT_DISABLE_NONE 
      | PwmEmios_0/PwmEmiosChannels_9/EmiosChPhaseShift - 0 
      | PwmEmios_0/PwmEmiosChannels_9/EmiosChPrescaler - EMIOS_PWM_IP_CLOCK_DIV_1 
      | PwmEmios_0/PwmEmiosChannels_9/EmiosChPrescalerAlternate - EMIOS_PWM_IP_CLOCK_DIV_1 
      | PwmEmios_0/PwmEmiosChannels_9/EmiosChPrescalerSource - EMIOS_PWM_IP_PS_SRC_MODULE_CLOCK 
      | PwmEmios_0/PwmEmiosChannels_9/EmiosChTrigger - 0 
      | PwmEmios_0/PwmEmiosChannels_9/Index - 0 
      | PwmEmios_0/PwmEmiosChannels_9/PwmEmiosBusRef - /Mcl/Mcl/MclConfig/EmiosCommon_0/EmiosMclMasterBus_0 
      | PwmEmios_0/PwmHwInstance - Emios_0 
      | PwmEmios_1/Index - 1 
      | PwmEmios_1/PwmEmiosChannels - PwmEmiosChannels_0 PwmEmiosChannels_1 PwmEmiosChannels_19 PwmEmiosChannels_20 PwmEmiosChannels_21 PwmEmiosChannels_22 
      | PwmEmios_1/PwmEmiosChannels_0/EmiosChCounterBus - EMIOS_PWM_IP_BUS_A 
      | PwmEmios_1/PwmEmiosChannels_0/EmiosChDeadtime - 0 
      | PwmEmios_1/PwmEmiosChannels_0/EmiosChFlagGeneration - Trailing_Edge 
      | PwmEmios_1/PwmEmiosChannels_0/EmiosChFreeze - false 
      | PwmEmios_1/PwmEmiosChannels_0/EmiosChId - CH_0 
      | PwmEmios_1/PwmEmiosChannels_0/EmiosChInterrupt - EMIOS_PWM_IP_INTERRUPT_REQUEST 
      | PwmEmios_1/PwmEmiosChannels_0/EmiosChMode - EMIOS_PWM_IP_MODE_OPWMB 
      | PwmEmios_1/PwmEmiosChannels_0/EmiosChOutputDisable - EMIOS_PWM_IP_OUTPUT_DISABLE_NONE 
      | PwmEmios_1/PwmEmiosChannels_0/EmiosChPhaseShift - 0 
      | PwmEmios_1/PwmEmiosChannels_0/EmiosChPrescaler - EMIOS_PWM_IP_CLOCK_DIV_1 
      | PwmEmios_1/PwmEmiosChannels_0/EmiosChPrescalerAlternate - EMIOS_PWM_IP_CLOCK_DIV_1 
      | PwmEmios_1/PwmEmiosChannels_0/EmiosChPrescalerSource - EMIOS_PWM_IP_PS_SRC_MODULE_CLOCK 
      | PwmEmios_1/PwmEmiosChannels_0/EmiosChTrigger - 0 
      | PwmEmios_1/PwmEmiosChannels_0/Index - 2 
      | PwmEmios_1/PwmEmiosChannels_0/PwmEmiosBusRef - /Mcl/Mcl/MclConfig/EmiosCommon_1/EmiosMclMasterBus_0 
      | PwmEmios_1/PwmEmiosChannels_1/EmiosChCounterBus - EMIOS_PWM_IP_BUS_A 
      | PwmEmios_1/PwmEmiosChannels_1/EmiosChDeadtime - 0 
      | PwmEmios_1/PwmEmiosChannels_1/EmiosChFlagGeneration - Trailing_Edge 
      | PwmEmios_1/PwmEmiosChannels_1/EmiosChFreeze - false 
      | PwmEmios_1/PwmEmiosChannels_1/EmiosChId - CH_1 
      | PwmEmios_1/PwmEmiosChannels_1/EmiosChInterrupt - EMIOS_PWM_IP_INTERRUPT_REQUEST 
      | PwmEmios_1/PwmEmiosChannels_1/EmiosChMode - EMIOS_PWM_IP_MODE_OPWMB 
      | PwmEmios_1/PwmEmiosChannels_1/EmiosChOutputDisable - EMIOS_PWM_IP_OUTPUT_DISABLE_NONE 
      | PwmEmios_1/PwmEmiosChannels_1/EmiosChPhaseShift - 0 
      | PwmEmios_1/PwmEmiosChannels_1/EmiosChPrescaler - EMIOS_PWM_IP_CLOCK_DIV_1 
      | PwmEmios_1/PwmEmiosChannels_1/EmiosChPrescalerAlternate - EMIOS_PWM_IP_CLOCK_DIV_1 
      | PwmEmios_1/PwmEmiosChannels_1/EmiosChPrescalerSource - EMIOS_PWM_IP_PS_SRC_MODULE_CLOCK 
      | PwmEmios_1/PwmEmiosChannels_1/EmiosChTrigger - 0 
      | PwmEmios_1/PwmEmiosChannels_1/Index - 3 
      | PwmEmios_1/PwmEmiosChannels_1/PwmEmiosBusRef - /Mcl/Mcl/MclConfig/EmiosCommon_1/EmiosMclMasterBus_0 
      | PwmEmios_1/PwmEmiosChannels_19/EmiosChCounterBus - EMIOS_PWM_IP_BUS_A 
      | PwmEmios_1/PwmEmiosChannels_19/EmiosChDeadtime - 0 
      | PwmEmios_1/PwmEmiosChannels_19/EmiosChFlagGeneration - Trailing_Edge 
      | PwmEmios_1/PwmEmiosChannels_19/EmiosChFreeze - false 
      | PwmEmios_1/PwmEmiosChannels_19/EmiosChId - CH_19 
      | PwmEmios_1/PwmEmiosChannels_19/EmiosChInterrupt - EMIOS_PWM_IP_INTERRUPT_REQUEST 
      | PwmEmios_1/PwmEmiosChannels_19/EmiosChMode - EMIOS_PWM_IP_MODE_OPWMB 
      | PwmEmios_1/PwmEmiosChannels_19/EmiosChOutputDisable - EMIOS_PWM_IP_OUTPUT_DISABLE_NONE 
      | PwmEmios_1/PwmEmiosChannels_19/EmiosChPhaseShift - 0 
      | PwmEmios_1/PwmEmiosChannels_19/EmiosChPrescaler - EMIOS_PWM_IP_CLOCK_DIV_1 
      | PwmEmios_1/PwmEmiosChannels_19/EmiosChPrescalerAlternate - EMIOS_PWM_IP_CLOCK_DIV_1 
      | PwmEmios_1/PwmEmiosChannels_19/EmiosChPrescalerSource - EMIOS_PWM_IP_PS_SRC_MODULE_CLOCK 
      | PwmEmios_1/PwmEmiosChannels_19/EmiosChTrigger - 0 
      | PwmEmios_1/PwmEmiosChannels_19/Index - 0 
      | PwmEmios_1/PwmEmiosChannels_19/PwmEmiosBusRef - /Mcl/Mcl/MclConfig/EmiosCommon_1/EmiosMclMasterBus_0 
      | PwmEmios_1/PwmEmiosChannels_20/EmiosChCounterBus - EMIOS_PWM_IP_BUS_A 
      | PwmEmios_1/PwmEmiosChannels_20/EmiosChDeadtime - 0 
      | PwmEmios_1/PwmEmiosChannels_20/EmiosChFlagGeneration - Trailing_Edge 
      | PwmEmios_1/PwmEmiosChannels_20/EmiosChFreeze - false 
      | PwmEmios_1/PwmEmiosChannels_20/EmiosChId - CH_20 
      | PwmEmios_1/PwmEmiosChannels_20/EmiosChInterrupt - EMIOS_PWM_IP_INTERRUPT_REQUEST 
      | PwmEmios_1/PwmEmiosChannels_20/EmiosChMode - EMIOS_PWM_IP_MODE_OPWMB 
      | PwmEmios_1/PwmEmiosChannels_20/EmiosChOutputDisable - EMIOS_PWM_IP_OUTPUT_DISABLE_NONE 
      | PwmEmios_1/PwmEmiosChannels_20/EmiosChPhaseShift - 0 
      | PwmEmios_1/PwmEmiosChannels_20/EmiosChPrescaler - EMIOS_PWM_IP_CLOCK_DIV_1 
      | PwmEmios_1/PwmEmiosChannels_20/EmiosChPrescalerAlternate - EMIOS_PWM_IP_CLOCK_DIV_1 
      | PwmEmios_1/PwmEmiosChannels_20/EmiosChPrescalerSource - EMIOS_PWM_IP_PS_SRC_MODULE_CLOCK 
      | PwmEmios_1/PwmEmiosChannels_20/EmiosChTrigger - 0 
      | PwmEmios_1/PwmEmiosChannels_20/Index - 1 
      | PwmEmios_1/PwmEmiosChannels_20/PwmEmiosBusRef - /Mcl/Mcl/MclConfig/EmiosCommon_1/EmiosMclMasterBus_0 
      | PwmEmios_1/PwmEmiosChannels_21/EmiosChCounterBus - EMIOS_PWM_IP_BUS_A 
      | PwmEmios_1/PwmEmiosChannels_21/EmiosChDeadtime - 0 
      | PwmEmios_1/PwmEmiosChannels_21/EmiosChFlagGeneration - Trailing_Edge 
      | PwmEmios_1/PwmEmiosChannels_21/EmiosChFreeze - false 
      | PwmEmios_1/PwmEmiosChannels_21/EmiosChId - CH_21 
      | PwmEmios_1/PwmEmiosChannels_21/EmiosChInterrupt - EMIOS_PWM_IP_INTERRUPT_REQUEST 
      | PwmEmios_1/PwmEmiosChannels_21/EmiosChMode - EMIOS_PWM_IP_MODE_OPWMB 
      | PwmEmios_1/PwmEmiosChannels_21/EmiosChOutputDisable - EMIOS_PWM_IP_OUTPUT_DISABLE_NONE 
      | PwmEmios_1/PwmEmiosChannels_21/EmiosChPhaseShift - 0 
      | PwmEmios_1/PwmEmiosChannels_21/EmiosChPrescaler - EMIOS_PWM_IP_CLOCK_DIV_1 
      | PwmEmios_1/PwmEmiosChannels_21/EmiosChPrescalerAlternate - EMIOS_PWM_IP_CLOCK_DIV_1 
      | PwmEmios_1/PwmEmiosChannels_21/EmiosChPrescalerSource - EMIOS_PWM_IP_PS_SRC_MODULE_CLOCK 
      | PwmEmios_1/PwmEmiosChannels_21/EmiosChTrigger - 0 
      | PwmEmios_1/PwmEmiosChannels_21/Index - 4 
      | PwmEmios_1/PwmEmiosChannels_21/PwmEmiosBusRef - /Mcl/Mcl/MclConfig/EmiosCommon_1/EmiosMclMasterBus_0 
      | PwmEmios_1/PwmEmiosChannels_22/EmiosChCounterBus - EMIOS_PWM_IP_BUS_A 
      | PwmEmios_1/PwmEmiosChannels_22/EmiosChDeadtime - 0 
      | PwmEmios_1/PwmEmiosChannels_22/EmiosChFlagGeneration - Trailing_Edge 
      | PwmEmios_1/PwmEmiosChannels_22/EmiosChFreeze - false 
      | PwmEmios_1/PwmEmiosChannels_22/EmiosChId - CH_22 
      | PwmEmios_1/PwmEmiosChannels_22/EmiosChInterrupt - EMIOS_PWM_IP_INTERRUPT_REQUEST 
      | PwmEmios_1/PwmEmiosChannels_22/EmiosChMode - EMIOS_PWM_IP_MODE_OPWMB 
      | PwmEmios_1/PwmEmiosChannels_22/EmiosChOutputDisable - EMIOS_PWM_IP_OUTPUT_DISABLE_NONE 
      | PwmEmios_1/PwmEmiosChannels_22/EmiosChPhaseShift - 0 
      | PwmEmios_1/PwmEmiosChannels_22/EmiosChPrescaler - EMIOS_PWM_IP_CLOCK_DIV_1 
      | PwmEmios_1/PwmEmiosChannels_22/EmiosChPrescalerAlternate - EMIOS_PWM_IP_CLOCK_DIV_1 
      | PwmEmios_1/PwmEmiosChannels_22/EmiosChPrescalerSource - EMIOS_PWM_IP_PS_SRC_MODULE_CLOCK 
      | PwmEmios_1/PwmEmiosChannels_22/EmiosChTrigger - 0 
      | PwmEmios_1/PwmEmiosChannels_22/Index - 5 
      | PwmEmios_1/PwmEmiosChannels_22/PwmEmiosBusRef - /Mcl/Mcl/MclConfig/EmiosCommon_1/EmiosMclMasterBus_0 
      | PwmEmios_1/PwmHwInstance - Emios_1 
      | PwmEmios_2/Index - 2 
      | PwmEmios_2/PwmEmiosChannels - PwmEmiosChannels_7 
      | PwmEmios_2/PwmEmiosChannels_7/EmiosChCounterBus - EMIOS_PWM_IP_BUS_A 
      | PwmEmios_2/PwmEmiosChannels_7/EmiosChDeadtime - 0 
      | PwmEmios_2/PwmEmiosChannels_7/EmiosChFlagGeneration - Trailing_Edge 
      | PwmEmios_2/PwmEmiosChannels_7/EmiosChFreeze - false 
      | PwmEmios_2/PwmEmiosChannels_7/EmiosChId - CH_7 
      | PwmEmios_2/PwmEmiosChannels_7/EmiosChInterrupt - EMIOS_PWM_IP_INTERRUPT_REQUEST 
      | PwmEmios_2/PwmEmiosChannels_7/EmiosChMode - EMIOS_PWM_IP_MODE_OPWMB 
      | PwmEmios_2/PwmEmiosChannels_7/EmiosChOutputDisable - EMIOS_PWM_IP_OUTPUT_DISABLE_NONE 
      | PwmEmios_2/PwmEmiosChannels_7/EmiosChPhaseShift - 0 
      | PwmEmios_2/PwmEmiosChannels_7/EmiosChPrescaler - EMIOS_PWM_IP_CLOCK_DIV_2 
      | PwmEmios_2/PwmEmiosChannels_7/EmiosChPrescalerAlternate - EMIOS_PWM_IP_CLOCK_DIV_2 
      | PwmEmios_2/PwmEmiosChannels_7/EmiosChPrescalerSource - EMIOS_PWM_IP_PS_SRC_MODULE_CLOCK 
      | PwmEmios_2/PwmEmiosChannels_7/EmiosChTrigger - 0 
      | PwmEmios_2/PwmEmiosChannels_7/Index - 0 
      | PwmEmios_2/PwmEmiosChannels_7/PwmEmiosBusRef - /Mcl/Mcl/MclConfig/EmiosCommon_2/EmiosMclMasterBus_0 
      | PwmEmios_2/PwmHwInstance - Emios_2 
      | PwmEtpu - PwmChannelConfigSet 
      | PwmGeneral - PwmGeneral 
      | PwmGeneral/PwmDevErrorDetect - true 
      | PwmGeneral/PwmDutycycleUpdatedEndperiod - false 
      | PwmGeneral/PwmEnableDualClockMode - false 
      | PwmGeneral/PwmEnableUserModeSupport - false 
      | PwmGeneral/PwmIndex - 0 
      | PwmGeneral/PwmMultiChannelSync - false 
      | PwmGeneral/PwmMultipartitionEnabled - false 
      | PwmGeneral/PwmNotificationSupported - true 
      | PwmGeneral/PwmPeriodUpdatedEndperiod - true
      settings: SourceProductName=NXP Model-Based Design Toolbox for S32K3 MCUs
  HsdDriveCommand Struct1 : MATLAB Function  TreatAsAtomicUnit=on
  Json编码器 : Subsystem
  MATLAB Function : MATLAB Function  TreatAsAtomicUnit=on
  MATLAB Function1 : MATLAB Function  TreatAsAtomicUnit=on
  RGBLED0state : DataStoreMemory  DataStoreName=RGBLED0state  WriteAfterWriteMsg=warning  InitialValue=[0 0 0]  ShowAdditionalParam=off  OutDataTypeStr=uint8
  RT : RateTransition
  RT1 : RateTransition  OutPortSampleTime=0.05
  Signal Specification1 : SignalSpecification  Dimensions=8
  Step : Step  Commented=on
  Step1 : Step  Commented=on
  Step2 : Step  Time=3
  Subsystem : Subsystem
  Subsystem1 : Subsystem
  Subsystem10 : Subsystem
  Subsystem11 : Subsystem
  Subsystem12 : Subsystem
  Subsystem13 : Subsystem
  Subsystem2 : Subsystem
  Subsystem5 : Subsystem  Commented=on
  Subsystem6 : Subsystem  TreatAsAtomicUnit=on
      settings: RTWSystemCode=Nonreusable function
  Subsystem7 : Subsystem
  Subsystem8 : Subsystem
  Subsystem9 : Subsystem  Commented=on
  Terminator{,1..8} (9 alike) : Terminator
  Uart1 : mbd_s32k3_cdd_library/Uart  api_func=Uart_AsyncReceive  channel=UartChannel_0  baudrate=UART_BAUDRATE_1200  transfer_type=UART_SEND  timeout=0  text=<binary blob, 5810 chars, not shown>
      settings: SourceProductName=NXP Model-Based Design Toolbox for S32K3 MCUs
  指令报文解码器 : Subsystem  TreatAsAtomicUnit=on
      settings: RTWSystemCode=Nonreusable function
  控制状态机 : Subsystem  Commented=on
  无线调试模式管理子系统 : Subsystem
  核心状态信息发送 : Subsystem
  输出3s初始化 : Subsystem  Commented=on
  错误码数据发送(未) : Subsystem
  错误码数据发送(未)1 : Subsystem
  wires:
  [Task_50ms_BatsAnalyze] -> Subsystem6/Trigger
  [Task_10ms_DrsDrive] -> Subsystem8/Trigger
  [Task_1000ms_Indicator] -> Subsystem7/Trigger
  Bus Creator1/1 -> Delay/1
  Hardware_Interrupt_Handler4/6 -> Bus Creator1/2  "Length"
  Constant6/1 -> Bus Creator1/3  "Remote"
  [Task_50ms_HsdDrive] -> HSD驱动子系统/Trigger
  Hardware_Interrupt_Handler4/1 -> 指令报文解码器/Trigger
  Delay/1 -> 指令报文解码器/1(In1)
  [Task_50ms_HsdDiagnose] -> HSD诊断分析子系统/Trigger
  Constant13/1 -> Bus Creator1/4  "Error"
  Hardware_Interrupt_Handler4/4 -> Bitwise AND/1  "ID"
  [DrsDriveCommand] -> Subsystem8/1(In5)
  Constant4/1 -> Bus Creator1/1  "Extended"
  Data Type Conversion2/1 -> Bus Creator1/6  "Timestamp"
  Hardware_Interrupt_Handler4/5 -> Signal Specification1/1  "Data"
  Hardware_Interrupt_Handler/2 -> Terminator/1
  [Task_1000ms_DebugManage] -> 无线调试模式管理子系统/Trigger
  Step/1 -> Subsystem9/Trigger
  Hardware_Interrupt_Handler1/1 -> Subsystem1/Trigger
  Uart1/2 -> Terminator1/1
  Constant1/1 -> Uart1/1
  Uart1/1 -> Subsystem10/1(In1)
  Hardware_Interrupt_Handler/3 -> 4G通信控制状态机1/1(signal)  "2:接收事件"
  Bitwise AND/1 -> Bus Creator1/5  "ID"
  Hardware_Interrupt_Handler4/2 -> Terminator2/1
  Signal Specification1/1 -> Bus Creator1/7
  Hardware_Interrupt_Handler4/3 -> Terminator4/1
  Constant/1 -> Data Type Conversion2/1
  [BatsData] -> Json编码器/1(In2)  "Bus_Vbats_Data"
  [HsdDiagnoseResult] -> Json编码器/2(In11)
  [HsdDiagnoseValue] -> Json编码器/3(In12)
  [VehicleData] -> Json编码器/4(In1)
  Hardware_Interrupt_Handler2/1 -> Subsystem11/Trigger
  Hardware_Interrupt_Handler5/1 -> Subsystem12/Trigger
  Subsystem6/2(Out2) -> [BatsData]
  HSD诊断分析子系统/2(Out2) -> [HsdDiagnoseResult]
  HSD诊断分析子系统/1(Out1) -> [HsdDiagnoseValue]
  RT1/1 -> [HsdDriveCommandsCAN]
  HsdDriveCommand Struct1/1(HsdDriveCommandsInit) -> 指令报文解码器/2(HsdDriveCommandsInit)
  [BatsData] -> 核心状态信息发送/1(In1)
  RT/1 -> [VehicleData]
  Subsystem10/1(Out1) -> Terminator3/1
  Subsystem10/2(Out2) -> Terminator5/1
  Subsystem10/3(Out3) -> Terminator6/1
  MATLAB Function/1(DiagnoseValueStruct) -> HSD诊断分析子系统/1(DiagnoseValueStruct)
  MATLAB Function1/1(DiagnoseResultStruct) -> HSD诊断分析子系统/2(DiagnoseResultStruct)
  指令报文解码器/2(DrsDriveCommand) -> [DrsDriveCommand]
  [DrsDriveCommand] -> 核心状态信息发送/2(In2)
  [Task_1000ms_CanMsgSend1] -> 核心状态信息发送/Trigger
  [Task_1000ms_CanMsgSend2] -> 错误码数据发送(未)/Trigger
  指令报文解码器/3(VehicleData) -> RT/1
  指令报文解码器/1(HsdDriveCommands) -> RT1/1
  4G通信控制状态机1/1(output) -> Subsystem2/1(output)
  Constant2/1 -> 4G通信控制状态机1/2(enable)
  Json编码器/1(stringin) -> 4G通信控制状态机1/3(stringin)
  Hardware_Interrupt_Handler/1 -> Terminator7/1  "rx_event"
  [Task_1000ms_MqttPublish] -> 4G通信控制状态机1/Trigger
  Function-Call Split/4 -> [Task_1000ms_CanMsgSend1]
  Function-Call Split/5 -> [Task_1000ms_CanMsgSend2]
  Function-Call Split1/3 -> [Task_50ms_BatsAnalyze]
  10ms1/1 -> [Task_10ms_DrsDrive]
  Function-Call Split1/2 -> [Task_50ms_HsdDrive]
  50ms1/1 -> Function-Call Split1/1
  1000ms1/1 -> Function-Call Split/1
  Function-Call Split/1 -> [Task_1000ms_Indicator]
  Function-Call Split/3 -> [Task_1000ms_MqttPublish]
  Function-Call Split/2 -> [Task_1000ms_DebugManage]
  Function-Call Split1/1 -> [Task_50ms_HsdDiagnose]
  [HsdDriveCommandsCAN] -> Subsystem13/2(In2)
  Step2/1 -> Subsystem13/1(In1)
  Subsystem13/1(y1) -> HSD驱动子系统/1(y)
  Subsystem6/1(RbcmCoreData) -> Terminator8/1
  Step1/1 -> Subsystem5/1(In1)
  1000ms4/1 -> 输出3s初始化/Trigger
  [Task_1000ms_CanMsgSend3] -> 错误码数据发送(未)1/Trigger
  Function-Call Split/6 -> [Task_1000ms_CanMsgSend3]
